simulink model "adaptation_MRAC_control"  (R2017a)
settings: Solver=VariableStepAuto  StartTime=0.0  StopTime=tf  RelTol=1e-3
undefined symbols (not defined in the file or in its folder): A_p, A_r, adaptationfun, ahat_0, B_p, B_r, C_p, C_r, controlfun, D_p, D_r, reffun, x_0, xr_0
settings Model: Creator=bruno  LastModifiedBy=bruno

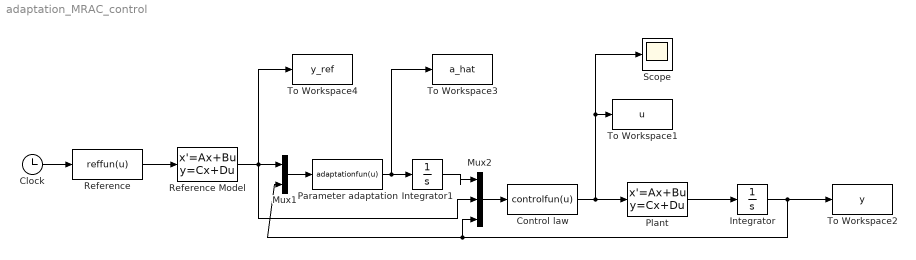
== system adaptation_MRAC_control ==
  Clock : Clock
  Control law : MATLABFcn  MATLABFcn=controlfun(u)  OutputSignalType=real
  Integrator : Integrator  InitialCondition=x_0
  Integrator1 : Integrator  InitialCondition=ahat_0
  Mux1 : Mux  Inputs=2
  Mux2 : Mux  Inputs=3
  Parameter adaptation : MATLABFcn  MATLABFcn=adaptationfun(u)  OutputSignalType=real
  Plant : StateSpace  A=A_p  B=B_p  C=C_p  D=D_p  X0=x_0
  Reference : MATLABFcn  MATLABFcn=reffun(u)  OutputSignalType=real
  Reference Model : StateSpace  A=A_r  B=B_r  C=C_r  D=D_r  X0=xr_0
  Scope : Scope
  To Workspace1 : ToWorkspace  VariableName=u  SaveFormat=Timeseries  SampleTime=-1
  To Workspace2 : ToWorkspace  VariableName=y  SaveFormat=Timeseries  SampleTime=-1
  To Workspace3 : ToWorkspace  VariableName=a_hat  SaveFormat=Timeseries  SampleTime=-1
  To Workspace4 : ToWorkspace  VariableName=y_ref  SaveFormat=Timeseries  SampleTime=-1
  wires:
  Integrator/1 -> Mux1/2, Mux2/3, To Workspace2/1
  Clock/1 -> Reference/1
  Mux1/1 -> Parameter adaptation/1
  Control law/1 -> Scope/1, To Workspace1/1, Plant/1
  Plant/1 -> Integrator/1
  Reference/1 -> Reference Model/1
  Parameter adaptation/1 -> Integrator1/1, To Workspace3/1
  Integrator1/1 -> Mux2/1
  Mux2/1 -> Control law/1
  Reference Model/1 -> To Workspace4/1, Mux2/2, Mux1/1
